simulink model "Load_NLMPC_GRU"  (R2023b)
settings: Solver=FixedStepAuto  StartTime=0.0  StopTime=10.0  FixedStep=0.1  RelTol=1e-3
libraries: vehdynlibviscommon x1, autolibshared x1, mpclib x1, robotcorelib x1, sim3dlib x1, sim3dautolib x1
settings Model: Creator=Arash  LastModifiedBy=Arash

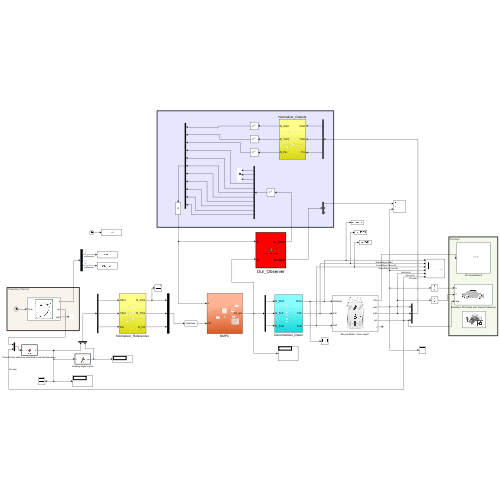
[thumbnail: Simulink's stored preview of the top-level diagram]
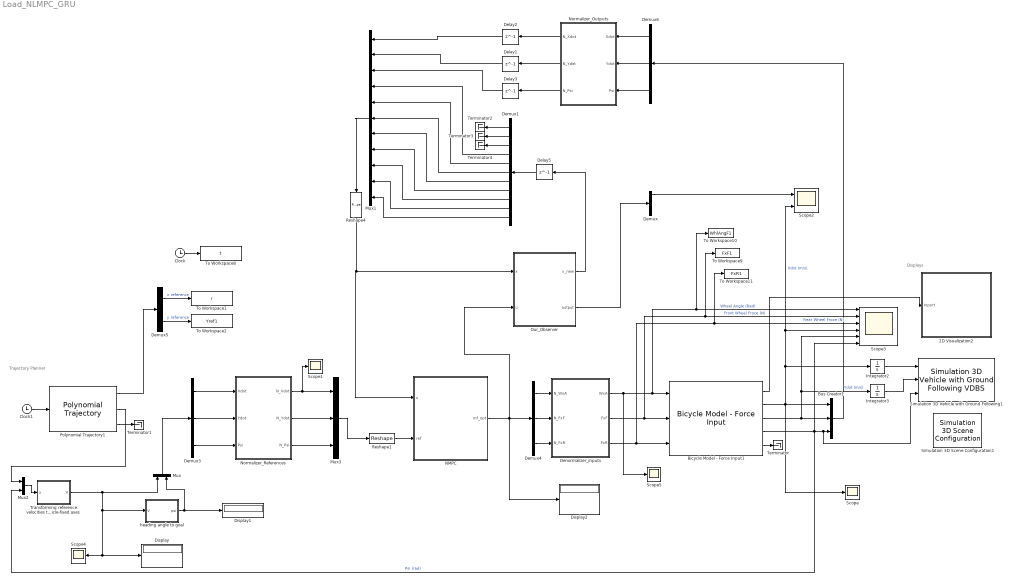
== system Load_NLMPC_GRU ==
  note: Trajectory Planner
  note: Displays
  2D Visualization2 : Subsystem
      mask Display: image("visualization.JPG");
  Bicycle Model - Force Input1 : autolibshared/Bicycle Model - Force Input  trackMode=Single (bicycle)  inputMode=External longitudinal forces  frontSteerMode=on  rearSteerMode=off  windMode=off  muMode=off  extFMode=off  extMMode=off  aMode=3  NF=1  NR=1  m=2000  a=1.4  b=1.6  h=0.35  X_o=0  xdot_o=0  CalphaMode=off  sigmaMode=on  w=[1.4,1.4]  Cy_f=12e3  Cy_r=11e3  sigma_f=.1  sigma_r=.1  alpha_f_brk=[-.1 .1]  Cy_f_data=[-9e3 9e3]  alpha_r_brk=[-.1 .1]  Cy_r_data=[-9e3 9e3]  Y_o=0  ydot_o=0  Izz=4000  psi_o=0  r_o=0  Af=2  Cd=.3  Cl=.1  Cpm=.1  beta_w=[0 0.01:0.01:0.3]  Cs=[0 0.01:0.01:0.3]  Cym=[0 1e-6:0.01:0.3]  Pabs=101325  Tair=273  g=9.81  mu=1  xdot_tol=.01  Fznom=5000  Fxtire_sat=1e6  Fytire_sat=1e6  longOff=0  latOff=0  vertOff=0
      settings: LibrarySourceBlock=drivingscenarioandsensors/Bicycle Model - Force Input
  Bus Creator1 : BusCreator  Inputs=3
  Clock : Clock
  Clock1 : Clock
      settings: Decimation=19
  Delay1 : Delay  DelayLength=1  InitialCondition=[0 0 0]
  Delay2 : Delay  DelayLength=1  InitialCondition=[0 0 0]
  Delay3 : Delay  DelayLength=1  InitialCondition=[0 0 0]
  Delay5 : Delay  DelayLength=1  InitialCondition=zeros(11,1)
  Demux{,3..4,6} (4 alike) : Demux  Outputs=3
  Demux1 : Demux  Outputs=11
  Demux5 : Demux  Outputs=2
  Denormalizer_inputs : Subsystem
  Display : Display
  Display1 : Display
  Display2 : Display
  Integrator2 : Integrator
  Integrator3 : Integrator
  Mux : Mux  Inputs=2
  Mux1 : Mux  Inputs=11
  Mux2 : Mux  Inputs=2
  Mux3 : Mux  Inputs=3
  NMPC : Subsystem
  Normalizer_Outputs : Subsystem
  Normalizer_References : Subsystem
  Our_Observer : MATLAB Function  TreatAsAtomicUnit=on
  Polynomial Trajectory1 : robotcorelib/Polynomial Trajectory  WaypointSource=Internal  Waypoints=[ 0,5,10; 0,0,0]  TimePoints=[ 0,5,10]  TimeInterval=[ 1, 4 ]  Method=Cubic Polynomial  ParameterSource=Internal  VelocityBoundaryCondition=zeros( 2, 3 )  AccelerationBoundaryCondition=zeros( 2, 5 )  SimulateUsing=Interpreted execution
  Reshape1 : Reshape  OutputDimensionality=Customize  OutputDimensions=[1,3]
  Reshape4 : Reshape  OutputDimensionality=Customize  OutputDimensions=[11,1]
  Scope{,1,4..5} (4 alike) : Scope
  Scope2 : Scope  NumInputPorts=2
  Scope3 : Scope  NumInputPorts=6
  Simulation 3D Scene Configuration1 : sim3dlib/Simulation 3D Scene Configuration  Priority=0  ProjectFormat=Default Scenes  SceneDesc=Straight road  ProjectName=C:\Program Files\MATLAB\R2023b\toolbox\shared\sim3d_projects\automotive_project_windows\UE\WindowsNoEditor\VehicleSimulation.exe  ScenePath=/Game/Maps/HwStrght  EnableOpenDRIVE=off  vehTagList={'Custom';'Scene Origin';'SimulinkVehicle2'}  vehTag=SimulinkVehicle2  FreeCameraInitialTranslation=[0, 0, 0]  FreeCameraDefaultInitialTranslation=[-6, 0, 2]  FreeCameraInitialRotation=[0, 0, 0]  FreeCameraDefaultInitialRotation=[0, -15, 0]  OpVisEn=off  Ts=0.1  EnableWindow=on  EnableRemoteAccess=off  EnableWeather=off  SunAltitude=40.0  SunAzimuth=90  clouds=10  wind=1  fog=0  rain=0  EnableGeospatial=off  OriginHeight=200  OriginLatitude=40.744652  OriginLongitude=-73.988864  MapStyle=Aerial  AdditionalAssetIDs=[]  UseAdvancedSunSky=off  SolarTime=11  TimeZone=-5  Day=21  Month=9  Year=2022  UseDaylightSavingTime=on  DSTStartDay=10  DSTStartMonth=3  DSTEndDay=3  DSTEndMonth=11  DSTSwitchHour=2  sensorTag=MainCamera2  sensorId=2  sensorName=MainCamera2  mountLoc=Origin  offsetFlag=off  tmountOffset=[0, 0, 0]  rmountOffset=[0, 0, 0]  HorizontalResolution=1280  VerticalResolution=720  HorizontalFOV=60  mountPoint=[0 0 0]  mountOrientation=[0 0 0]  aMode=aMode  ID=2  GeoTrigger=Inactive
  Simulation 3D Vehicle with Ground Following1 : sim3dautolib/Simulation 3D Vehicle with Ground Following VDBS  Priority=-1  PassVehMesh=Hatchback  MeshPath=/MathWorksSimulation/Vehicles/Muscle/Meshes/SK_MuscleCar.SK_MuscleCar  TrackWidth=1.9  WheelBase=3  WheelRadius=0.35  VehColor=Green  InitialPos=[0,0,0]  InitialRot=[0, 0, 0]  ActorName=SimulinkVehicle2  VehLightsControl=off  HeadlightColor=[ 1, 1, 1 ]  HighBeamIntensity=100000  LowBeamIntensity=60000  HighBeamConeAngle=1.22  LowBeamConeAngle=1.22  LeftHeadlightOrientation=[ 0, 0 ]  RightHeadlightOrientation=[ 0, 0 ]  BrakelightIntensity=200  ReverselightIntensity=500  SignallightIntensity=500  SignallightPeriod=1  SignalPulseWidth=50  SampleTime=-1  ActorType=SimulinkVehicle  ID=2  aMode=2  ActorTag=SimulinkVehicle2  CoordinateScheme=SAE
      settings: LibrarySourceBlock=vehdynlibsim3d/Simulation 3D Vehicle with Ground Following
  Terminator{,1..4} (5 alike) : Terminator
  To Workspace1 : ToWorkspace  VariableName=r  SampleTime=-1
      settings: Save2DSignal=2-D array (concatenate along first dimension)
  To Workspace10 : ToWorkspace  VariableName=WhlAngF1  SaveFormat=Timeseries  SampleTime=0.1
  To Workspace11 : ToWorkspace  VariableName=FxR1  SaveFormat=Timeseries  SampleTime=0.1
  To Workspace2 : ToWorkspace  VariableName=Yref1  SampleTime=-1
      settings: Save2DSignal=2-D array (concatenate along first dimension)
  To Workspace8 : ToWorkspace  VariableName=t  SaveFormat=Timeseries  SampleTime=-1
  To Workspace9 : ToWorkspace  VariableName=FxF1  SaveFormat=Timeseries  SampleTime=0.1
  "Transforming reference velocities to vehicle-fixed axes " : MATLAB Function  TreatAsAtomicUnit=on
  heading angle to goal : MATLAB Function  TreatAsAtomicUnit=on
  wires:
  Normalizer_Outputs/1(N_Xdot) -> Delay2/1
  Normalizer_Outputs/3(N_Psi) -> Delay3/1
  Demux6/2 -> Normalizer_Outputs/2(Ydot)
  Demux4/2 -> Denormalizer_inputs/2(N_FxF)
  Reshape1/1 -> NMPC/2(ref)
  Normalizer_References/3(N_Psi) -> Mux3/3
  Bicycle Model - Force Input1/5 -> Terminator/1
  Normalizer_Outputs/2(N_Ydot) -> Delay1/1
  Denormalizer_inputs/1(WxA) -> Scope5/1, To Workspace10/1, Scope3/1, Bicycle Model - Force Input1/1  "Wheel Angle (Rad)"
  "Transforming reference velocities to vehicle-fixed axes "/1(V) -> Display/1, Scope4/1, heading angle to goal/1(V), Mux/1
  Integrator2/1 -> Simulation 3D Vehicle with Ground Following1/1
  Denormalizer_inputs/3(FxR) -> To Workspace11/1, Scope3/3, Bicycle Model - Force Input1/3  "Rear Wheel Froce (N)"
  heading angle to goal/1(psi) -> Display1/1, Mux/2
  Demux5/2 -> To Workspace2/1  "y reference"
  Demux6/1 -> Normalizer_Outputs/1(Xdot)
  Polynomial Trajectory1/1 -> Demux5/1
  Bus Creator1/1 -> Demux6/1
  Bicycle Model - Force Input1/1 -> 2D Visualization2/1(Inport)
  Integrator3/1 -> Simulation 3D Vehicle with Ground Following1/2
  Bicycle Model - Force Input1/3 -> Scope3/5, Integrator3/1, Bus Creator1/2  "Ydot (m/s)"
  Demux5/1 -> To Workspace1/1  "x reference"
  Bicycle Model - Force Input1/2 -> Scope/1, Scope2/2, Scope3/4, Integrator2/1, Bus Creator1/1  "Xdot (m/s)"
  Demux6/3 -> Normalizer_Outputs/3(Psi)
  Polynomial Trajectory1/2 -> Mux2/1
  Clock1/1 -> Polynomial Trajectory1/1
  Mux/1 -> Demux3/1
  Polynomial Trajectory1/3 -> Terminator1/1
  NMPC/1(mf_opt) -> Demux4/1, Display2/1, Our_Observer/2(u)
  Mux2/1 -> "Transforming reference velocities to vehicle-fixed axes "/1(x)
  Bicycle Model - Force Input1/4 -> Mux2/2, Simulation 3D Vehicle with Ground Following1/3, Bus Creator1/3, Scope3/6  "Psi (rad)"
  Demux3/2 -> Normalizer_References/2(Ydot)
  Normalizer_References/1(N_Xdot) -> Mux3/1, Scope1/1
  Demux4/1 -> Denormalizer_inputs/1(N_WxA)
  Demux4/3 -> Denormalizer_inputs/3(N_FxR)
  Demux3/1 -> Normalizer_References/1(Xdot)
  Normalizer_References/2(N_Ydot) -> Mux3/2
  Mux3/1 -> Reshape1/1
  Denormalizer_inputs/2(FxF) -> To Workspace9/1, Scope3/2, Bicycle Model - Force Input1/2  "Front Wheel Froce (N)"
  Demux3/3 -> Normalizer_References/3(Psi)
  Delay1/1 -> Mux1/2
  Delay3/1 -> Mux1/3
  Mux1/1 -> Reshape4/1
  Our_Observer/2(output) -> Demux/1
  Demux/1 -> Scope2/1
  Clock/1 -> To Workspace8/1
  Our_Observer/1(x_new) -> Delay5/1
  Delay2/1 -> Mux1/1
  Delay5/1 -> Demux1/1
  Demux1/1 -> Terminator2/1
  Demux1/2 -> Terminator3/1
  Demux1/3 -> Terminator4/1
  Demux1/4 -> Mux1/4
  Demux1/5 -> Mux1/5
  Demux1/6 -> Mux1/6
  Demux1/7 -> Mux1/7
  Demux1/8 -> Mux1/8
  Demux1/9 -> Mux1/9
  Demux1/10 -> Mux1/10
  Demux1/11 -> Mux1/11
  Reshape4/1 -> NMPC/1(x), Our_Observer/1(x)

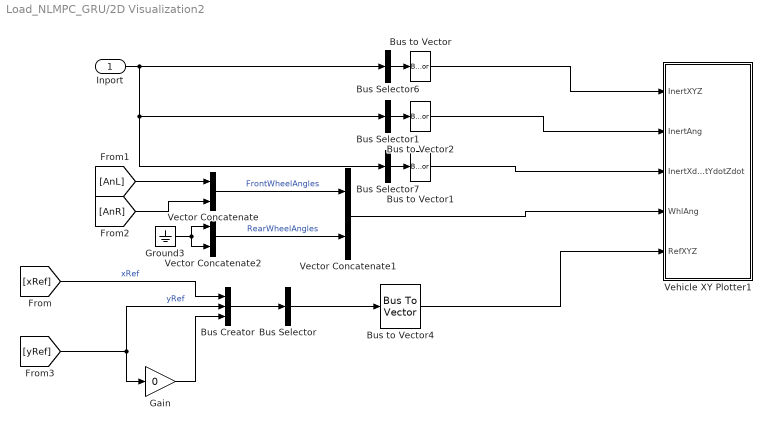
== system Load_NLMPC_GRU/2D Visualization2 ==
  Inport : Inport
  Bus Creator : BusCreator  Inputs=3
  Bus Selector : BusSelector  OutputSignals=xRef,yRef,signal3  OutputAsBus=on
  Bus Selector1 : BusSelector  OutputSignals=InertFrm.Cg.Ang.phi,InertFrm.Cg.Ang.theta,InertFrm.Cg.Ang.psi  OutputAsBus=on
  Bus Selector6 : BusSelector  OutputSignals=InertFrm.Geom.Disp.X,InertFrm.Geom.Disp.Y,InertFrm.Geom.Disp.Z  OutputAsBus=on
  Bus Selector7 : BusSelector  OutputSignals=InertFrm.Geom.Vel.Xdot,InertFrm.Geom.Vel.Ydot,InertFrm.Geom.Vel.Zdot  OutputAsBus=on
  Bus to Vector{,1..2,4} (4 alike) : BusToVector
  Gain : Gain  Gain=0
  Ground3 : Ground
  Vector Concatenate : Concatenate
  Vector Concatenate1 : Concatenate
  Vector Concatenate2 : Concatenate
  Vehicle XY Plotter1 : Subsystem  mask(Vehicle XY Plotter){extRef=on, extStats=off, extTireF=off, a=2, b=2, w=2, figBorder=10, bufferSize=1024, velNorm=5, tireFNorm=1000, pltDT=0.2}
      mask prompts: extRef "Plot path reference, extRef"; extStats "Display speed, RPM and Gear"; extTireF "Display tire forces"; a "Distance to front axle from CG, a [m]:"; b "Distance to rear axle from CG, b [m]:"; w "Track width, w [m]:"; figBorder "Distance to figure borders, figBorder [m]:"; bufferSize "Path buffer sampe size, bufferSize []:"; velNorm "Velocity vector scaling, velNorm [m*s/m]:"; tireFNorm "Tire force vector scaling, tireFNorm [m/N]:"; pltDT "Plot update rate, pltDT [s]:"
      mask help:
      | This block will display a MATLAB figure which indicates the vehicle path, current position and heading velocity.
      | An optional path reference is also provided.
      mask init:
      | block = gcb;
      | if autoblkschecksimstopped(block)
      |     ParamNames = {'extRef';'extStats';'extTireF';'extTireF'};
      |     PortNames = {'RefXYZ';'Stats';'TireFx';'TireFy'};
      |     for idx=1:length(PortNames)
      |         InportOption  = {'built-in/Ground', [PortNames{idx}, ' Ground'];...
      |             'built-in/Inport',PortNames{idx}};
      |         if ~strcmp(get_param(block,ParamNames{idx}),'on')
      |             NewBlkHdl = autoblksreplaceblock(block, InportOption, 1);
      |             set_param(NewBlkHdl, 'ShowName', 'off');
      |         else
      |             autoblksreplaceblock(block, InportOption, 2);
      |         end
      |     end
      |     InportNames = {'InertXYZ';'InertAng';'InertXdotYdotZdot';'WhlAng';'RefXYZ';'Stats';'TireFx';'TireFy'};
      |     FoundNames = get_param(find_system(block, 'LookUnderMasks', 'all', 'SearchDepth', 1, 'FollowLinks', 'on', 'BlockType', 'Inport'), 'Name');
      |     [~,PortI] = intersect(InportNames, FoundNames);
      |     PortI = sort(PortI);
      |     for idx = 1:length(PortI)
      |         set_param([block, '/', InportNames{PortI(idx)}], 'Port', num2str(idx));
      |     end
      | end
      mask TypeOptions a: Vehicle XY Plotter/a
      mask TypeOptions b: Vehicle XY Plotter/b
      mask TypeOptions w: Vehicle XY Plotter/w
      mask TypeOptions figBorder: Vehicle XY Plotter/figBorder
      mask TypeOptions bufferSize: Vehicle XY Plotter/bufferSize
      mask TypeOptions velNorm: Vehicle XY Plotter/velNorm
      mask TypeOptions tireFNorm: Vehicle XY Plotter/tireFNorm
      mask DialogControl Container3 Prompt: Plot and Display Options
  wires:
  Bus Creator/1 -> Bus Selector/1
  [xRef] -> Bus Creator/1  "xRef"
  Gain/1 -> Bus Creator/3
  [yRef] -> Gain/1, Bus Creator/2  "yRef"
  Bus Selector/1 -> Bus to Vector4/1
  Bus to Vector4/1 -> Vehicle XY Plotter1/5(RefXYZ)
  Inport/1 -> Bus Selector6/1, Bus Selector1/1, Bus Selector7/1
  [AnR] -> Vector Concatenate/2
  Bus Selector1/1 -> Bus to Vector2/1
  Bus to Vector2/1 -> Vehicle XY Plotter1/2(InertAng)
  Bus to Vector/1 -> Vehicle XY Plotter1/1(InertXYZ)
  Bus to Vector1/1 -> Vehicle XY Plotter1/3(InertXdotYdotZdot)
  Bus Selector7/1 -> Bus to Vector1/1
  Vector Concatenate2/1 -> Vector Concatenate1/2  "RearWheelAngles"
  [AnL] -> Vector Concatenate/1
  Vector Concatenate/1 -> Vector Concatenate1/1  "FrontWheelAngles"
  Bus Selector6/1 -> Bus to Vector/1
  Ground3/1 -> Vector Concatenate2/2, Vector Concatenate2/1
  Vector Concatenate1/1 -> Vehicle XY Plotter1/4(WhlAng)

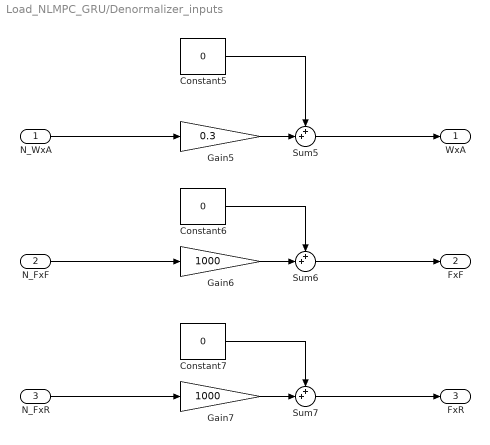
== system Load_NLMPC_GRU/Denormalizer_inputs ==
  N_WxA : Inport
  N_FxF : Inport  Port=2
  N_FxR : Inport  Port=3
  Constant5 : Constant  Value=0
  Constant6 : Constant  Value=0
  Constant7 : Constant  Value=0
  Gain5 : Gain  Gain=0.3
  Gain6 : Gain  Gain=1000
  Gain7 : Gain  Gain=1000
  Sum5 : Sum  Inputs=++|
  Sum6 : Sum  Inputs=++|
  Sum7 : Sum  Inputs=++|
  WxA : Outport
  FxF : Outport  Port=2
  FxR : Outport  Port=3
  wires:
  Sum6/1 -> FxF/1
  Gain7/1 -> Sum7/2
  Gain5/1 -> Sum5/2
  Constant7/1 -> Sum7/1
  Gain6/1 -> Sum6/2
  Sum5/1 -> WxA/1
  Constant5/1 -> Sum5/1
  Constant6/1 -> Sum6/1
  Sum7/1 -> FxR/1
  N_FxR/1 -> Gain7/1
  N_WxA/1 -> Gain5/1
  N_FxF/1 -> Gain6/1

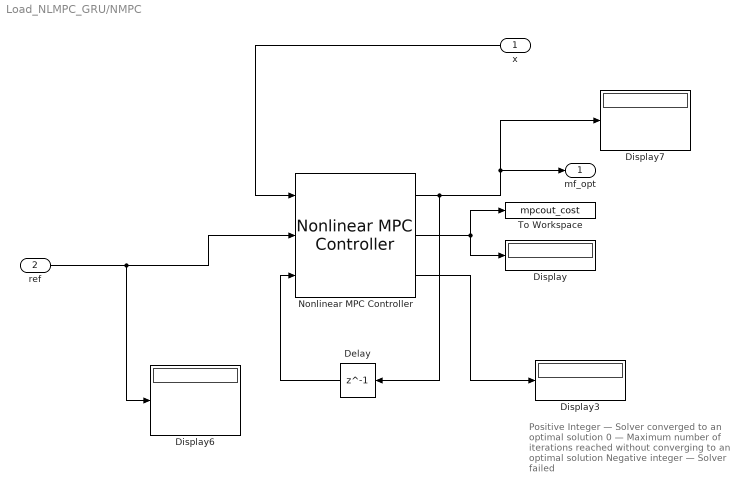
== system Load_NLMPC_GRU/NMPC ==
  note: Positive Integer — Solver converged to an optimal solution
      | 0 — Maximum number of iterations reached without converging to an optimal solution
      | Negative integer — Solver failed
  x : Inport
  ref : Inport  Port=2
  Delay : Delay  DelayLength=1  InitialCondition=[0 0 0]
  Display{,3,6..7} (4 alike) : Display
  Nonlinear MPC Controller : mpclib/Nonlinear MPC Controller  SCDEnableBlockLinearizationSpecification=on  nlmpcobj=nlobj  UseObjectTs=on  UseMEX=off  md_enabled=off  mvtarget_enabled=off  param_enabled=off  cost_enabled=on  mvseq_enabled=off  stateseq_enabled=off  ovseq_enabled=off  slack_enabled=off  status_enabled=on  ov_min=off  ov_max=off  mv_min=off  mv_max=off  mvrate_min=off  mvrate_max=off  state_min=off  state_max=off  ov_weight=off  mv_weight=off  mvrate_weight=off  ecr_weight=off  nlp_initialize=off
  To Workspace : ToWorkspace  VariableName=mpcout_cost  SaveFormat=Timeseries  SampleTime=-1
  mf_opt : Outport
  wires:
  Nonlinear MPC Controller/1 -> Delay/1, Display7/1, mf_opt/1
  x/1 -> Nonlinear MPC Controller/1
  ref/1 -> Nonlinear MPC Controller/2, Display6/1
  Nonlinear MPC Controller/2 -> Display/1, To Workspace/1
  Nonlinear MPC Controller/3 -> Display3/1
  Delay/1 -> Nonlinear MPC Controller/3

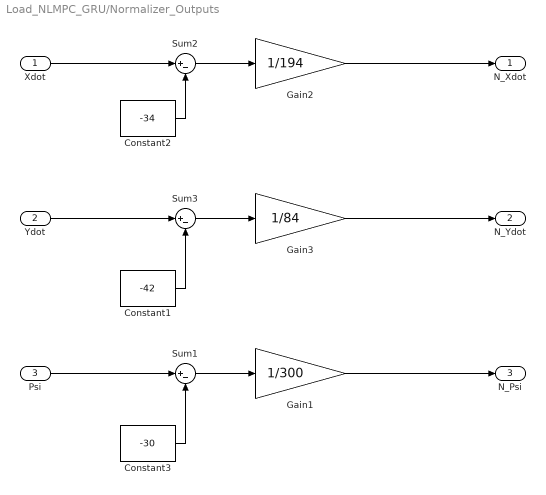
== system Load_NLMPC_GRU/Normalizer_Outputs ==
  Xdot : Inport
  Ydot : Inport  Port=2
  Psi : Inport  Port=3
  Constant1 : Constant  Value=-42
  Constant2 : Constant  Value=-34
  Constant3 : Constant  Value=-30
  Gain1 : Gain  Gain=1/300
  Gain2 : Gain  Gain=1/194
  Gain3 : Gain  Gain=1/84
  Sum1 : Sum  Inputs=|+-
  Sum2 : Sum  Inputs=|+-
  Sum3 : Sum  Inputs=|+-
  N_Xdot : Outport
  N_Ydot : Outport  Port=2
  N_Psi : Outport  Port=3
  wires:
  Gain2/1 -> N_Xdot/1
  Sum3/1 -> Gain3/1
  Constant2/1 -> Sum2/2
  Gain3/1 -> N_Ydot/1
  Constant1/1 -> Sum3/2
  Sum2/1 -> Gain2/1
  Xdot/1 -> Sum2/1
  Ydot/1 -> Sum3/1
  Sum1/1 -> Gain1/1
  Gain1/1 -> N_Psi/1
  Constant3/1 -> Sum1/2
  Psi/1 -> Sum1/1

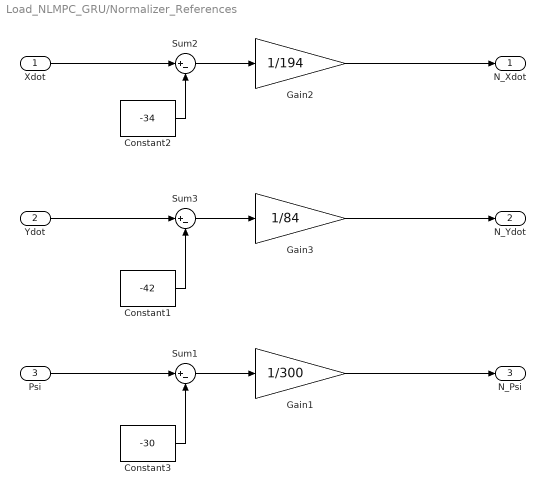
== system Load_NLMPC_GRU/Normalizer_References ==
  Xdot : Inport
  Ydot : Inport  Port=2
  Psi : Inport  Port=3
  Constant1 : Constant  Value=-42
  Constant2 : Constant  Value=-34
  Constant3 : Constant  Value=-30
  Gain1 : Gain  Gain=1/300
  Gain2 : Gain  Gain=1/194
  Gain3 : Gain  Gain=1/84
  Sum1 : Sum  Inputs=|+-
  Sum2 : Sum  Inputs=|+-
  Sum3 : Sum  Inputs=|+-
  N_Xdot : Outport
  N_Ydot : Outport  Port=2
  N_Psi : Outport  Port=3
  wires:
  Gain2/1 -> N_Xdot/1
  Sum3/1 -> Gain3/1
  Constant2/1 -> Sum2/2
  Gain3/1 -> N_Ydot/1
  Constant1/1 -> Sum3/2
  Sum2/1 -> Gain2/1
  Xdot/1 -> Sum2/1
  Ydot/1 -> Sum3/1
  Sum1/1 -> Gain1/1
  Gain1/1 -> N_Psi/1
  Constant3/1 -> Sum1/2
  Psi/1 -> Sum1/1

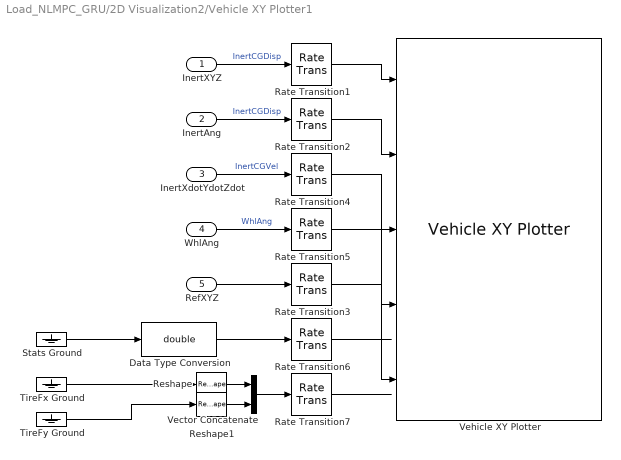
== system Load_NLMPC_GRU/2D Visualization2/Vehicle XY Plotter1 ==
  InertXYZ : Inport
  InertAng : Inport  Port=2
  InertXdotYdotZdot : Inport  Port=3
  WhlAng : Inport  Port=4
  RefXYZ : Inport  Port=5
  Data Type Conversion : DataTypeConversion  OutDataTypeStr=double  SaturateOnIntegerOverflow=off  RndMeth=Floor
  Rate Transition{1..7} (7 alike) : RateTransition  Deterministic=off  OutPortSampleTime=pltDT
  Reshape : Reshape  OutputDimensionality=Row vector (2-D)
  Reshape1 : Reshape  OutputDimensionality=Row vector (2-D)
  Stats Ground : Ground
  TireFx Ground : Ground
  TireFy Ground : Ground
  Vector Concatenate : Concatenate  Mode=Multidimensional array
  Vehicle XY Plotter : vehdynlibviscommon/Vehicle XY Plotter  w=w  a=a  b=b  figBorder=figBorder  bufferSize=bufferSize  extStats=off  extTireF=off
  wires:
  TireFy Ground/1 -> Reshape1/1
  TireFx Ground/1 -> Reshape/1
  Stats Ground/1 -> Data Type Conversion/1
  InertAng/1 -> Rate Transition2/1  "InertCGDisp"
  InertXdotYdotZdot/1 -> Rate Transition4/1  "InertCGVel"
  InertXYZ/1 -> Rate Transition1/1  "InertCGDisp"
  WhlAng/1 -> Rate Transition5/1  "WhlAng"
  Rate Transition3/1 -> Vehicle XY Plotter/5
  Rate Transition1/1 -> Vehicle XY Plotter/1
  Rate Transition2/1 -> Vehicle XY Plotter/2
  Rate Transition4/1 -> Vehicle XY Plotter/3
  Rate Transition5/1 -> Vehicle XY Plotter/4
  Rate Transition6/1 -> ?
  Data Type Conversion/1 -> Rate Transition6/1
  Rate Transition7/1 -> ?
  RefXYZ/1 -> Rate Transition3/1
  Reshape/1 -> Vector Concatenate/1
  Reshape1/1 -> Vector Concatenate/2
  Vector Concatenate/1 -> Rate Transition7/1

== matlab function Load_NLMPC_GRU/Our_Observer ==
  data: x input; x_new output; u input; output output
function [x_new, output]   =  GRU_function(x,u)
h_t  =  x(4 : end);
% Initialize weights and biases
W_input  =  [-0.095897 -0.012435 0.027793 0.371231 -0.005094 0.124832;-0.001613 0.000280 -0.001032 0.120837 -0.051541 -0.089163;-0.020829 0.003020 0.000128 -0.006392 0.119840 -0.011985;0.028522 -0.010024 -0.006695 -0.344397 -0.163646 -0.246519;-0.014741 -0.006104 -0.004543 0.112781 -0.026581 -0.000932;-0.007655 0.006522 0.001021 -0.541686 -0.135704 -0.007165;0.037126 0.004060 0.002918 0.086177 0.001136 0.029026;0.002731 -0.000119 -0.000031 0.041135 -0.030265 0.003032;-0.303361 -0.174777 0.058984 -1.088399 -0.456023 -0.266408;-0.682596 0.071107 -0.007277 -1.080279 -0.588972 -0.674350;-0.492108 -0.059440 0.044719 0.031613 -0.562382 -0.583926;-0.108377 -0.227406 -0.161012 -0.701523 0.055240 -0.152693;-0.120685 -0.201047 -0.488457 -0.981044 -0.293663 -0.192205;-0.091291 -0.368637 -0.245565 -0.688684 -0.521099 -0.461413;-0.052068 -0.011567 -0.023209 0.221322 0.022841 -0.018732;-0.465640 -0.004387 -0.037150 -0.965176 -0.472427 -0.608690;-0.013075 -0.021464 -0.008653 0.443277 0.355848 0.100046;0.008791 0.008809 0.004294 0.418115 -0.046355 -0.381566;0.078418 -0.003842 0.010197 0.153296 -0.005085 -0.137296;0.029651 0.026241 0.015859 -0.127482 0.100388 0.586224;-0.028239 -0.037358 -0.032341 -0.221630 0.039616 -0.224430;-0.075767 0.007184 -0.007589 -0.021942 0.567109 -0.033828;-0.055810 0.077036 0.047819 -0.022970 -0.067335 0.124617;0.055425 0.009086 0.011745 -0.309683 0.625754 -0.110820;];
W_recurrent  =  [0.449549 0.025030 -0.096241 -0.168294 -0.235541 0.000154 -0.286506 -0.000000;-0.000000 0.000000 0.004807 0.000000 -0.000000 0.064231 -0.000000 0.024651;0.485105 0.052874 0.000033 -0.027222 -0.000000 0.376345 -0.000000 -0.000000;0.001067 -0.000073 -0.000000 0.094900 -0.001176 0.090062 0.000000 -0.052772;-0.000014 0.000096 0.070818 -0.000116 -0.001819 -0.000000 0.000021 -0.031904;-0.075881 -0.059038 -0.000000 -0.009897 -0.000000 -0.000000 -0.001961 0.022182;0.000000 -0.037331 -0.000000 -0.000000 -0.000632 -0.000009 0.000667 -0.000000;-0.078798 -0.000033 -0.011031 -0.000003 0.000052 0.000000 0.000000 0.032599;-0.573147 0.000000 0.151396 -0.000011 1.082723 -0.816462 0.652375 -0.000000;-0.382626 -0.000039 0.008461 -0.253424 0.018146 -0.200148 1.273786 0.000000;-0.021385 -0.000000 0.498021 -0.297493 0.368878 -0.457074 0.526535 -0.050971;-0.005362 -0.231979 -0.010862 -0.000000 0.009229 0.000005 0.252313 0.447642;-0.108325 -0.144418 0.031101 -0.000121 0.296174 -0.068469 0.285247 -0.000000;-0.101816 -0.000001 0.268416 -0.000000 0.414597 -0.267433 0.478665 0.000000;-0.057857 0.000000 0.033577 0.000008 0.090569 -0.000002 0.054693 0.012192;-0.064325 -0.120602 0.000030 -0.259008 0.775705 -0.380701 0.572294 -0.004287;0.000000 0.000000 0.000000 -0.000000 0.001459 -0.000000 0.004608 -0.000000;-0.016701 -0.094781 -0.000000 -0.000000 0.000000 -0.000000 0.000000 0.022603;-0.011072 -0.006802 -0.003487 -0.000000 0.000000 -0.159166 0.000000 -0.018679;-0.099606 0.000000 0.005900 -0.273327 0.001836 -0.000673 0.005513 -0.000001;-0.000000 -0.000000 0.019067 0.000004 -0.000000 -0.000000 -0.000000 -0.246290;-0.083940 -0.000000 0.000559 0.003144 0.011304 -0.000065 0.002755 -0.023331;-0.000002 -0.000000 0.090047 -0.000000 0.017483 -0.000001 0.000000 -0.003226;0.000002 0.000000 0.034014 0.000005 0.000000 -0.000000 0.000416 -0.058670;];

W_dense  = [0.792528 0.899694 0.410716 0.321609 -0.486353 0.538735 -0.320163 -0.824348;0.928638 0.112599 -0.479506 0.023697 0.092886 0.233405 0.061675 1.027291;0.620761 -0.762181 -0.405004 1.095673 -0.361138 -0.155618 -0.394896 -0.451011;];


bias  =  [0.066898;0.135457;0.237060;0.274518;0.456006;0.272725;0.185509;-0.027074;-1.068504;-0.939111;-1.220924;-0.671026;-1.704713;-0.605181;-0.165316;-1.658573;-0.092363;-0.071420;0.068987;0.003822;-0.087872;0.075973;-0.021838;0.016971;0.066898;0.135457;0.237060;0.274518;0.456006;0.272725;0.185509;-0.027074;-1.068504;-0.939111;-1.220924;-0.671026;-1.704713;-0.605181;-0.165316;-1.658573;-0.262571;-0.034982;0.072780;-0.067652;0.011298;0.081524;-0.047508;0.006683;];

b_dense = [0.111769;0.219248;0.135490;];


%% Given shapes
W_is  =  size(W_input,1)/3;
W_rs  =  size(W_recurrent);
bias_shape  =  size(bias);
input_shape  =  size(u);

W_r = W_input(1 : W_is, : );
W_z = W_input(W_is + 1 : 2*W_is, : );
W_h = W_input(2*W_is + 1 : end, : );

R_r = W_recurrent(1 : W_is, : );
R_z = W_recurrent(W_is + 1 : 2*W_is, : );
R_h = W_recurrent(2*W_is + 1 : end, : );

BW_r = bias(1 : W_is, : );
BW_z = bias(W_is + 1 : 2*W_is, : );
BW_h = bias(2*W_is + 1 : 3*W_is, : );

BR_r = bias(3*W_is + 1 : 4*W_is, : );
BR_z = bias(4*W_is + 1 : 5*W_is, : );
BR_h = bias(5*W_is + 1 : end, : );

% Initialize hidden state
%h_t =  zeros(W_rs,1);

%Reset Gate
r_t  =  sigmoid(W_r*u + R_r*h_t + BW_r + BR_r);
%Update Gate
z_t  =  sigmoid(W_z*u + R_z*h_t + BW_z + BR_z);

% Candidate State
h_t_hat  =  tanh(W_h*u + r_t.*(R_h*h_t  + BR_h) + BW_h);

% s1 = size(z_t)
% s2 = size(h_t_hat)
% s3 = size(h_t)

% Hidden State
h_t = (1-z_t).*h_t_hat + z_t.*h_t;

% Apply activation function
out_gru  =  h_t;

% Fully connected Layer
output  =  W_dense*out_gru  +  b_dense;

x_new  =  [output(1, : ); output(2, : );output(3, : ); h_t];

== matlab function Load_NLMPC_GRU/heading angle to goal ==
  data: V input; psi output
function psi = fcn(V)

v1 =V(1);
v2 =V(2);
psi = atan2(v2,v1);

== matlab function Load_NLMPC_GRU/Transforming reference velocities to vehicle-fixed axes  ==
  data: x input; V output
function V = fcn(x)


V = [cos(x(3)) sin(x(3));
    -sin(x(3)) cos(x(3))]*[x(1); x(2)];
